simulink model "DiscreteRedOrd"  (R2020b)
settings: Solver=FixedStepAuto  StartTime=0.0  StopTime=3  FixedStep=1e-4  RelTol=1e-4
undefined symbols (not defined in the file): daq, drv, gbox, mech, mld, mot, rads2rpm, rpm2rads, sens, sim, state_space, tustin
settings Model: Creator=Utente  LastModifiedBy=Utente

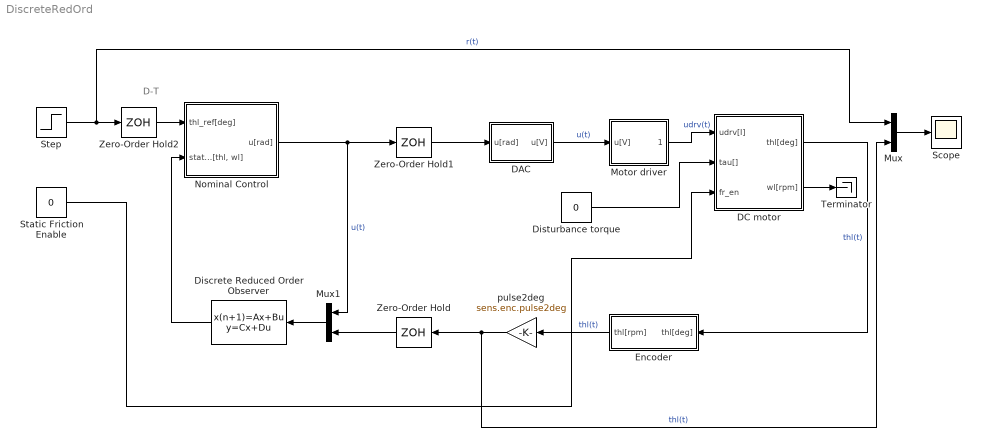
== system DiscreteRedOrd ==
  note: D-T
  DAC : Subsystem
  DC motor : Subsystem
  Discrete Reduced Order Observer : DiscreteStateSpace  A=tustin.Phi  B=tustin.Gam  C=tustin.H  D=tustin.J  SampleTime=sim.T_samp
  Disturbance torque : Constant  Value=0
  Encoder : Subsystem
  Motor driver : Subsystem
  Mux : Mux  Inputs=2
  Mux1 : Mux  Inputs=2
  Nominal Control : Subsystem
  Scope : Scope
  Static Friction Enable : Constant  Value=0
  Step : Step  Time=0  After=50  SampleTime=0
  Terminator : Terminator
  Zero-Order Hold : ZeroOrderHold  SampleTime=sim.T_samp
  Zero-Order Hold1 : ZeroOrderHold  SampleTime=sim.T_samp
  Zero-Order Hold2 : ZeroOrderHold  SampleTime=sim.T_samp
  pulse2deg : Gain  Gain=sens.enc.pulse2deg
  wires:
  Step/1 -> Zero-Order Hold2/1, Mux/1  "r(t)"
  DC motor/1(thl[deg]) -> Encoder/1(thl[deg])  "thl(t)"
  Nominal Control/1(u[rad]) -> Mux1/1, Zero-Order Hold1/1  "u(t)"
  Mux/1 -> Scope/1
  Encoder/1(thl[rpm]) -> pulse2deg/1  "thl(t)"
  Mux1/1 -> Discrete Reduced Order Observer/1
  DC motor/2(wl[rpm]) -> Terminator/1
  pulse2deg/1 -> Mux/2, Zero-Order Hold/1  "thl(t)"
  Zero-Order Hold/1 -> Mux1/2
  Zero-Order Hold1/1 -> DAC/1(u[rad])
  DAC/1(u[V]) -> Motor driver/1(u[V])  "u(t)"
  Motor driver/1(udrv[I]) -> DC motor/1(udrv[I])  "udrv(t)"
  Disturbance torque/1 -> DC motor/2(tau[])
  Static Friction Enable/1 -> DC motor/3(fr_en)
  Discrete Reduced Order Observer/1 -> Nominal Control/2("state[thl, wl]")
  Zero-Order Hold2/1 -> Nominal Control/1(thl_ref[deg])

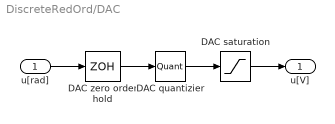
== system DiscreteRedOrd/DAC ==
  u[rad] : Inport
  DAC quantizier : Quantizer  QuantizationInterval=daq.dac.q
  DAC saturation : Saturate  UpperLimit=daq.dac.vdd  LowerLimit=daq.dac.vss
  DAC zero order hold : ZeroOrderHold  SampleTime=daq.dac.T_s
  u[V] : Outport
  wires:
  DAC quantizier/1 -> DAC saturation/1
  DAC zero order hold/1 -> DAC quantizier/1
  DAC saturation/1 -> u[V]/1
  u[rad]/1 -> DAC zero order hold/1

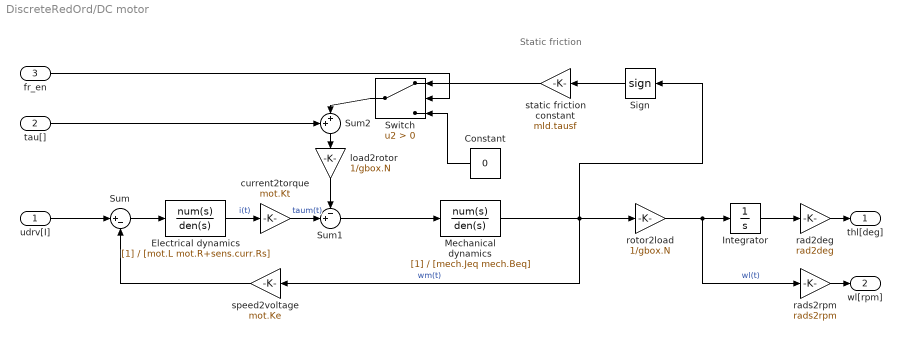
== system DiscreteRedOrd/DC motor ==
  note: Static friction
  udrv[I] : Inport  Unit=V
  tau[] : Inport  Port=2  Unit=V
  fr_en : Inport  Port=3  Unit=V
  Constant : Constant  Value=0
  Electrical dynamics : TransferFcn  Denominator=[mot.L mot.R+sens.curr.Rs]
  Integrator : Integrator
  Mechanical dynamics : TransferFcn  Denominator=[mech.Jeq mech.Beq]
  Sign : Signum  ZeroCross=off
  Sum : Sum  Inputs=|+-
  Sum1 : Sum  Inputs=-+|
  Sum2 : Sum  Inputs=++|
  Switch : Switch  Criteria=u2 > Threshold
  current2torque : Gain  Gain=mot.Kt
  load2rotor : Gain  Gain=1/gbox.N
  rad2deg : Gain  Gain=rad2deg
  rads2rpm : Gain  Gain=rads2rpm
  rotor2load : Gain  Gain=1/gbox.N
  speed2voltage : Gain  Gain=mot.Ke
  static friction constant : Gain  Gain=mld.tausf
  thl[deg] : Outport  Unit=deg
  wl[rpm] : Outport  Port=2  Unit=rpm
  wires:
  load2rotor/1 -> Sum1/1
  Mechanical dynamics/1 -> Sign/1, rotor2load/1, speed2voltage/1  "wm(t)"
  Sign/1 -> static friction constant/1
  current2torque/1 -> Sum1/2  "taum(t)"
  Sum1/1 -> Mechanical dynamics/1
  speed2voltage/1 -> Sum/2
  rotor2load/1 -> rads2rpm/1, Integrator/1  "wl(t)"
  Electrical dynamics/1 -> current2torque/1  "i(t)"
  Integrator/1 -> rad2deg/1
  Sum/1 -> Electrical dynamics/1
  rads2rpm/1 -> wl[rpm]/1
  rad2deg/1 -> thl[deg]/1
  udrv[I]/1 -> Sum/1
  Sum2/1 -> load2rotor/1
  tau[]/1 -> Sum2/1
  static friction constant/1 -> Switch/1
  Switch/1 -> Sum2/2
  Constant/1 -> Switch/3
  fr_en/1 -> Switch/2

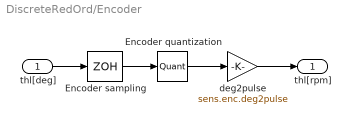
== system DiscreteRedOrd/Encoder ==
  thl[deg] : Inport
  Encoder quantization : Quantizer  QuantizationInterval=sens.enc.q
  Encoder sampling : ZeroOrderHold  SampleTime=sens.enc.T_s
  deg2pulse : Gain  Gain=sens.enc.deg2pulse
  thl[rpm] : Outport
  wires:
  Encoder quantization/1 -> deg2pulse/1
  deg2pulse/1 -> thl[rpm]/1
  Encoder sampling/1 -> Encoder quantization/1
  thl[deg]/1 -> Encoder sampling/1

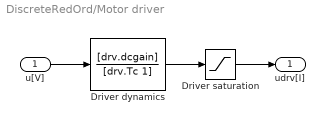
== system DiscreteRedOrd/Motor driver ==
  u[V] : Inport
  Driver dynamics : TransferFcn  Numerator=[drv.dcgain]  Denominator=[drv.Tc 1]
  Driver saturation : Saturate  UpperLimit=drv.vp  LowerLimit=drv.vm
  udrv[I] : Outport
  wires:
  Driver saturation/1 -> udrv[I]/1
  Driver dynamics/1 -> Driver saturation/1
  u[V]/1 -> Driver dynamics/1

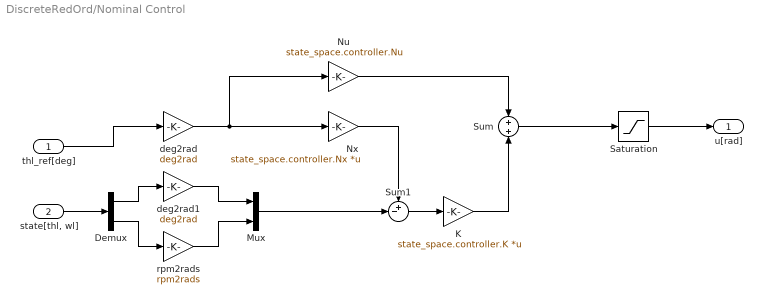
== system DiscreteRedOrd/Nominal Control ==
  thl_ref[deg] : Inport
  "state[thl, wl]" : Inport  Port=2
  Demux : Demux  Outputs=2
  K : Gain  Gain=state_space.controller.K  Multiplication=Matrix(K*u)
  Mux : Mux  Inputs=2
  Nu : Gain  Gain=state_space.controller.Nu
  Nx : Gain  Gain=state_space.controller.Nx  Multiplication=Matrix(K*u)
  Saturation : Saturate  UpperLimit=daq.dac.vdd  LowerLimit=daq.dac.vss
  Sum : Sum  Inputs=+|+
  Sum1 : Sum  Inputs=+-|
  deg2rad : Gain  Gain=deg2rad
  deg2rad1 : Gain  Gain=deg2rad
  rpm2rads : Gain  Gain=rpm2rads
  u[rad] : Outport
  wires:
  rpm2rads/1 -> Mux/2
  thl_ref[deg]/1 -> deg2rad/1
  deg2rad1/1 -> Mux/1
  Saturation/1 -> u[rad]/1
  Demux/1 -> deg2rad1/1
  Sum/1 -> Saturation/1
  Demux/2 -> rpm2rads/1
  "state[thl, wl]"/1 -> Demux/1
  K/1 -> Sum/2
  deg2rad/1 -> Nx/1, Nu/1
  Nu/1 -> Sum/1
  Sum1/1 -> K/1
  Mux/1 -> Sum1/2
  Nx/1 -> Sum1/1
